simulink model "Example_2"  (R2017b)
settings: Solver=VariableStepAuto  StartTime=0.0  StopTime=30  RelTol=1e-3
libraries: simulink x1
settings Model: Creator=hoang  LastModifiedBy=hoang

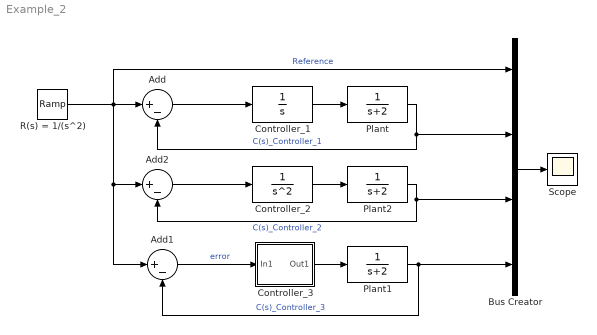
== system Example_2 ==
  Add : Sum  Inputs=|+-
  Add1 : Sum  Inputs=|+-
  Add2 : Sum  Inputs=|+-
  Bus Creator : BusCreator  Inputs=4
  Controller_1 : TransferFcn  Denominator=[1 0]
  Controller_2 : TransferFcn  Denominator=[1 0 0]
  Controller_3 : Subsystem
  Plant : TransferFcn  Denominator=[1 2]
  Plant1 : TransferFcn  Denominator=[1 2]
  Plant2 : TransferFcn  Denominator=[1 2]
  R(s) = 1/(s^2) : simulink/Sources/Ramp  slope=1  start=0  X0=0
  Scope : Scope
  wires:
  Controller_1/1 -> Plant/1
  Add/1 -> Controller_1/1
  Plant/1 -> Add/2, Bus Creator/2  "C(s)_Controller_1"
  Bus Creator/1 -> Scope/1
  Plant1/1 -> Bus Creator/4, Add1/2  "C(s)_Controller_3"
  R(s) = 1/(s^2)/1 -> Add1/1, Add2/1, Bus Creator/1, Add/1  "Reference"
  Add1/1 -> Controller_3/1(In1)  "error"
  Controller_3/1(Out1) -> Plant1/1
  Add2/1 -> Controller_2/1
  Controller_2/1 -> Plant2/1
  Plant2/1 -> Add2/2, Bus Creator/3  "C(s)_Controller_2"

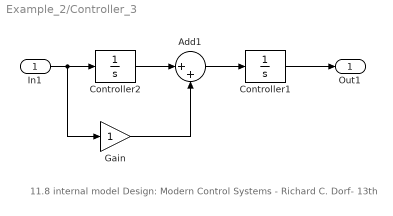
== system Example_2/Controller_3 ==
  note: 11.8 internal model Design: Modern Control Systems - Richard C. Dorf- 13th
  In1 : Inport
  Add1 : Sum  Inputs=|++
  Controller1 : TransferFcn  Denominator=[1 0]
  Controller2 : TransferFcn  Denominator=[1 0]
  Gain : Gain
  Out1 : Outport
  wires:
  In1/1 -> Gain/1, Controller2/1
  Controller1/1 -> Out1/1
  Controller2/1 -> Add1/1
  Add1/1 -> Controller1/1
  Gain/1 -> Add1/2
